simulink model "IEEE24bus_simplified"  (R2019b)
settings: Solver=ode23tb  StartTime=0.0  StopTime=100  MaxStep=1/60  RelTol=1e-4  AbsTol=1e-3  EnableMultiTasking=on
PreLoadFcn:
  | RTS96_data
values from neighbouring files (symbols this model uses):
  Efmax = 5    [IEEE24_bus.m]    (also in IEEE24bus_simplified_benchmark.m)
  Efmin = -5    [IEEE24_bus.m]    (also in IEEE24bus_simplified_benchmark.m)
  EXc_sys = [     0.06  25  0.2    0.0505  0.5685   0 0   0.091  0.35 ... (first row only)    [IEEE24bus_simplified_benchmark.m]
  FH1 = 12    [IEEE24bus_simplified_benchmark.m]
  FI1 = .9    (= 0.9)    [IEEE24bus_simplified_benchmark.m]
  FL1 = .1    (= 0.1)    [IEEE24bus_simplified_benchmark.m]
  KH1 = 100    [IEEE24bus_simplified_benchmark.m]
  KI1 = 1    [IEEE24_bus.m]    (also in IEEE24bus_simplified_benchmark.m = 20)
  KL1 = 10    [IEEE24bus_simplified_benchmark.m]
undefined symbols (not defined in the file or in its folder): D1, Delta
libraries: powerlib x157, sps_avr x11, powerlib_extras x1
(part 1 of 3)
settings Model: Creator=bx6353  LastModifiedBy=mingj
settings SolverCC: AutoScaleAbsTol=off  ZeroCrossControl=DisableAll
settings DataIOCC: InitialState=xFinal  LimitDataPoints=on  SaveFinalState=on  SaveFormat=Array  SignalLoggingSaveFormat=ModelDataLogs  ReturnWorkspaceOutputs=off
settings OptimizationCC: ExpressionDepthLimit=2147483647  InitFltsAndDblsToZero=on  LifeSpan=inf
settings DebuggingCC: SaveWithParameterizedLinksMsg=none  UnderspecifiedInitializationDetection=Classic  MergeDetectMultiDrivingBlocksExec=none  SignalResolutionControl=TryResolveAllWithWarning  SolverPrmCheckMsg=warning  MultiTaskDSMMsg=warning  MultiTaskCondExecSysMsg=none  FcnCallInpInsideContextMsg=warning  UnconnectedInputMsg=none  UnconnectedOutputMsg=none  UnconnectedLineMsg=none  StateNameClashWarn=warning  StrictBusMsg=ErrorOnBusTreatedAsVector  SFUnexpectedBacktrackingDiag=warning  SFNoUnconditionalDefaultTransitionDiag=warning  SFExecutionAtInitializationDiag=none  ArithmeticOperatorsInVariantConditions=warning
settings HardwareCC: ProdBitPerPointer=32  ProdBitPerSizeT=32  ProdBitPerPtrDiffT=32  ProdLargestAtomicFloat=None  ProdIntDivRoundTo=Undefined  ProdEndianess=Unspecified  ProdWordSize=32  ProdHWDeviceType=32-bit Generic
settings ModelReferenceCC: PropagateSignalLabelsOutOfModel=off
settings SFSimCC: SimUseLocalCustomCode=off  CustomCodeUndefinedFunction=UseInterfaceOnly
settings RTWCC: RTWUseLocalCustomCode=off
settings CodeAppCC: StateflowObjectComments=on
settings GRTTargetCC: TargetFcnLib=ansi_tfl_tmw.mat  TargetLangStandard=C89/C90 (ANSI)  GeneratePreprocessorConditionals=Disable all  CombineOutputUpdateFcns=off  GRTInterface=on
settings ConfigComp: CovMetricSettings=dw  CovHtmlReporting=on  CovSaveCumulativeToWorkspaceVar=on  CovSaveSingleToWorkspaceVar=on  CovExternalEMLEnable=off
settings SimscapeCC: SimscapeNormalizeSystem=off

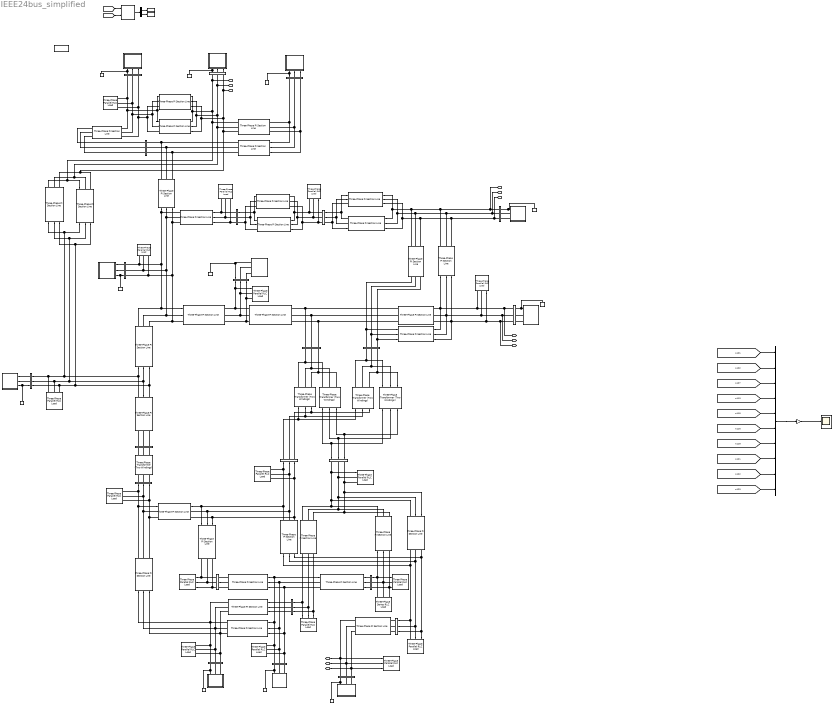
== system IEEE24bus_simplified ==
  101 : Subsystem
  102 : Subsystem
  107 : Subsystem
  113 : Subsystem
  114 : Subsystem
  115 : Subsystem
  116 : Subsystem
  118 : Subsystem
  121 : Subsystem
  122 : Subsystem
  123 : Subsystem
  3-phase  Instantaneous  Active & Reactive Power : powerlib_extras/Measurements/3-phase  Instantaneous  Active & Reactive Power
      settings: SourceProductName=Simscape Electrical  SourceProductBaseCode=PS
  A1 : powerlib/Elements/Three-Phase PI Section Line  LConnTagsString=a|b|c  RConnTagsString=A|B|C  Frequency=60  Resistances=[ 0.003*(138e3)^2/100e6*[1 3]]  Inductances=[ 0.014*(138e3)^2/(120*pi*100e6)*[1 3]]  Capacitances=[0.461*100e6/(120*pi*(138e3)^2)*[1 1/3]]  Length=1
      settings: SourceProductName=Simscape Electrical
  A10 : powerlib/Elements/Three-Phase PI Section Line  LConnTagsString=a|b|c  RConnTagsString=A|B|C  Frequency=60  Resistances=[ 0.014*(138e3)^2/100e6*[1 3]]  Inductances=[ 0.061*(138e3)^2/(120*pi*100e6)*[1 3]]  Capacitances=[2.459*100e6/(120*pi*((138e3)^2))*[1 1/3]]  Length=1
      settings: SourceProductName=Simscape Electrical
  A11 : powerlib/Elements/Three-Phase PI Section Line  LConnTagsString=a|b|c  RConnTagsString=A|B|C  Frequency=60  Resistances=[ 0.016*(138e3)^2/100e6*[1 3]]  Inductances=[ 0.061*(138e3)^2/(120*pi*100e6) *[1 3]]  Capacitances=[0.017*100e6/(120*pi*(138e3)^2) *[1 1/3]]  Length=1
      settings: SourceProductName=Simscape Electrical
  A12-1 : powerlib/Elements/Three-Phase PI Section Line  LConnTagsString=a|b|c  RConnTagsString=A|B|C  Frequency=60  Resistances=[ 0.043*(138e3)^2/100e6 *[1 3]]  Inductances="[ 0.165*(138e3)^2/(120*pi*100e6)  *[1 3]]"  Capacitances=[0.045*100e6/(120*pi*(138e3)^2) *[1 1/3]]  Length=1
      settings: SourceProductName=Simscape Electrical
  A13-2 : powerlib/Elements/Three-Phase PI Section Line  LConnTagsString=a|b|c  RConnTagsString=A|B|C  Frequency=60  Resistances=[ 0.043*(138E3)^2/100E6*[1 3]]  Inductances=[ 0.165*(138e3)^2/(120*pi*100e6)*[1 3]]  Capacitances=[0.045*100e6/(120*pi*(138e3)^2)*[1 1/3]]  Length=1
      settings: SourceProductName=Simscape Electrical
  A{7,14..17} (5 alike) : powerlib/Elements/Three-Phase Transformer (Two Windings)  Winding1Connection=Y  Winding2Connection=Y  CoreType=Three single-phase transformers  SetSaturation=off  Hysteresis=off  DataFile='hysteresis'  SetInitialFlux=off  Measurements=None  UNITS=pu  NominalPower=[ 100e6 , 60 ]  Winding1=[ 230e3 , 0.001 , 0.084/2 ]  Winding2="[ 138e3 , 0.001 , 0.084/2  ]"  Rm=500  Lm=500  L0=0.5  Saturation=[ 0,0 ; 0.0024,1.2 ; 1.0,1.52 ]  InitialFluxes=[ 0.8 , -0.8 , 0.7 ]  BreakLoop=off  DiscreteSolver=Trapezoidal iterative  DataType=off  TransfoNumber=0
      settings: SourceProductName=Simscape Electrical
  A18 : powerlib/Elements/Three-Phase PI Section Line  LConnTagsString=a|b|c  RConnTagsString=A|B|C  Frequency=60  Resistances=[ 0.006*(230e3)^2/100e6*[1 3]]  Inductances=[ 0.048*(230e3)^2/(120*pi*100e6)*[1 3]]  Capacitances=[0.1*100e6/(120*pi*(230e3)^2)*[1 1/3]]  Length=1
      settings: SourceProductName=Simscape Electrical
  A19 : powerlib/Elements/Three-Phase PI Section Line  LConnTagsString=a|b|c  RConnTagsString=A|B|C  Frequency=60  Resistances=[ 0.005*(230e3)^2/(100e6)*[1 3]]  Inductances=[ 0.042*(230e3)^2/(120*pi*100e6)*[1 3]]  Capacitances=[0.088*100e6/(120*pi*(230e3)^2)*[1 1/3]]  Length=1
      settings: SourceProductName=Simscape Electrical
  A2 : powerlib/Elements/Three-Phase PI Section Line  LConnTagsString=a|b|c  RConnTagsString=A|B|C  Frequency=60  Resistances=[ 0.055*(138e3)^2/100e6*[1 3]]  Inductances=[ 0.211*(138e3)^2/(120*pi*100e6)*[1 3]]  Capacitances=[0.057*100e6/(120*pi*(138e3)^2) *[1 1/3]]  Length=1
      settings: SourceProductName=Simscape Electrical
  A20 : powerlib/Elements/Three-Phase PI Section Line  LConnTagsString=a|b|c  RConnTagsString=A|B|C  Frequency=60  Resistances=[ 0.006*(230e3)^2/100e6*[1 3]]  Inductances=[ 0.048*(230e3)^2/(120*pi*100e6)*[1 3]]  Capacitances=[0.1*100e6/(120*pi*(230e3)^2)*[1 1/3]]  Length=1
      settings: SourceProductName=Simscape Electrical
  A21 : powerlib/Elements/Three-Phase PI Section Line  LConnTagsString=a|b|c  RConnTagsString=A|B|C  Frequency=60  Resistances=[ 0.012*(230e3)^2/100e6*[1 3]]  Inductances=[ 0.097*(230e3)^2/(120*pi*100e6)*[1 3]]  Capacitances=[0.203*100e6/(120*pi*(230e3)^2)*[1 1/3]]  Length=1
      settings: SourceProductName=Simscape Electrical
  A22 : powerlib/Elements/Three-Phase PI Section Line  LConnTagsString=a|b|c  RConnTagsString=A|B|C  Frequency=60  Resistances=[ 0.011*(230e3)^2/100e6*[1 3]]  Inductances=[ 0.087*(230e3)^2/(120*pi*100e6) *[1 3]]  Capacitances=[0.182*100e6/(120*pi*(230e3)^2) *[1 1/3]]  Length=1
      settings: SourceProductName=Simscape Electrical
  A23 : powerlib/Elements/Three-Phase PI Section Line  LConnTagsString=a|b|c  RConnTagsString=A|B|C  Frequency=60  Resistances=[ 0.005*(230e3)^2/100e6*[1 3]]  Inductances=[ 0.059*(230e3)^2/(120*pi*100e6) *[1 3]]  Capacitances=[0.082*(100e6)/(120*pi*(230e3)^2)*[1 1/3]]  Length=1
      settings: SourceProductName=Simscape Electrical
  A24 : powerlib/Elements/Three-Phase PI Section Line  LConnTagsString=a|b|c  RConnTagsString=A|B|C  Frequency=60  Resistances=[ 0.002*(230e3)^2/100e6*[1 3]]  Inductances="[ 0.017*(230e3)^2/(120*pi*100e6)  *[1 3]]"  Capacitances=[0.036*100e6/(120*pi*(230e3)^2) *[1 1/3]]  Length=1
      settings: SourceProductName=Simscape Electrical
  A25-1 : powerlib/Elements/Three-Phase PI Section Line  LConnTagsString=a|b|c  RConnTagsString=A|B|C  Frequency=60  Resistances=[ 0.006*(230e3)^2/100e6*[1 3]]  Inductances=[ 0.049*(230e3)^2/(120*pi*100e6)*[1 3]]  Capacitances=[0.103*(100e6)/(120*pi*(230e3)^2)*[1 1/3]]  Length=1
      settings: SourceProductName=Simscape Electrical
  A25-2 : powerlib/Elements/Three-Phase PI Section Line  LConnTagsString=a|b|c  RConnTagsString=A|B|C  Frequency=60  Resistances=[ 0.006*(230e3)^2/100e6 *[1 3]]  Inductances=[ 0.049*(230e3)^2/(120*pi*100e6)*[1 3]]  Capacitances=[0.103*(100e6)/(120*pi*(230e3)^2)*[1 1/3]]  Length=1
      settings: SourceProductName=Simscape Electrical
  A26 : powerlib/Elements/Three-Phase PI Section Line  LConnTagsString=a|b|c  RConnTagsString=A|B|C  Frequency=60  Resistances=[ 0.007*(230e3)^2/100e6*[1 3]]  Inductances=[ 0.052*(230e3)^2/(120*pi*100e6) *[1 3]]  Capacitances=[0.109*100e6/(120*pi*(230e3)^2)*[1 1/3]]  Length=1
      settings: SourceProductName=Simscape Electrical
  A27 : powerlib/Elements/Three-Phase PI Section Line  LConnTagsString=a|b|c  RConnTagsString=A|B|C  Frequency=60  Resistances=[ 0.003*(230e3)^2/100e6*[1 3]]  Inductances=[ 0.026*(230e3)^2/(120*pi*100e6) *[1 3]]  Capacitances=[0.055*100e6/(120*pi*(230e3)^2) *[1 1/3]]  Length=1
      settings: SourceProductName=Simscape Electrical
  A28 : powerlib/Elements/Three-Phase PI Section Line  LConnTagsString=a|b|c  RConnTagsString=A|B|C  Frequency=60  Resistances=[ 0.003*(230e3)^2/100e6*[1 3]]  Inductances=[ 0.023*(230e3)^2/(120*pi*100e6)*[1 3]]  Capacitances=[0.049*100e6/(120*pi*(230e3)^2)*[1 1/3]]  Length=1
      settings: SourceProductName=Simscape Electrical
  A29 : powerlib/Elements/Three-Phase PI Section Line  LConnTagsString=a|b|c  RConnTagsString=A|B|C  Frequency=60  Resistances=[ 0.002*(230e3)^2/100e6*[1 3]]  Inductances=[ 0.014*(230e3)^2/(120*pi*100e6)*[1 3]]  Capacitances=[0.030*100e6/(120*pi*(230e3)^2)*[1 1/3]]  Length=1
      settings: SourceProductName=Simscape Electrical
  A3 : powerlib/Elements/Three-Phase PI Section Line  LConnTagsString=a|b|c  RConnTagsString=A|B|C  Frequency=60  Resistances=[0.022*(138e3)^2/100e6*[1 3]]  Inductances=[0.085*(138e3)^2/(120*pi*100e6)*[1 3]]  Capacitances=[0.023*100e6/(120*pi*(138e3)^2)*[1 1/3]]  Length=1
      settings: SourceProductName=Simscape Electrical
  A30 : powerlib/Elements/Three-Phase PI Section Line  LConnTagsString=a|b|c  RConnTagsString=A|B|C  Frequency=60  Resistances=[ 0.014*(230e3)^2/100e6 *[1 3]]  Inductances=[ 0.105*(230e3)^2/(120*pi*100e6) *[1 3]]  Capacitances=[0.221*100e6/(120*pi*(230e3)^2)*[1 1/3]]  Length=1
      settings: SourceProductName=Simscape Electrical
  A31-1 : powerlib/Elements/Three-Phase PI Section Line  LConnTagsString=a|b|c  RConnTagsString=A|B|C  Frequency=60  Resistances=[ 0.003*(230e3)^2/100e6*[1 3]]  Inductances=[ 0.026*(230e3)^2/(120*pi*100e6)*[1 3]]  Capacitances=[0.055*100e6/(120*pi*(230e3)^2)*[1 1/3]]  Length=1
      settings: SourceProductName=Simscape Electrical
  A31-2 : powerlib/Elements/Three-Phase PI Section Line  LConnTagsString=a|b|c  RConnTagsString=A|B|C  Frequency=60  Resistances=[ 0.003*(230e3)^2/100e6*[1 3]]  Inductances=[ 0.026*(230e3)^2/(120*pi*100e6) *[1 3]]  Capacitances=[0.055*100e6/(120*pi*(230e3)^2) *[1 1/3]]  Length=1
      settings: SourceProductName=Simscape Electrical
  A32-2 : powerlib/Elements/Three-Phase PI Section Line  LConnTagsString=a|b|c  RConnTagsString=A|B|C  Frequency=60  Resistances=[ 0.005*(230e3)^2/100e6 *[1 3]]  Inductances=[ 0.040*(230e3)^2/(120*pi*100e6)*[1 3]]  Capacitances=[0.083*100e6/(120*pi*(230e3)^2) *[1 1/3]]  Length=1
      settings: SourceProductName=Simscape Electrical
  A32-3 : powerlib/Elements/Three-Phase PI Section Line  LConnTagsString=a|b|c  RConnTagsString=A|B|C  Frequency=60  Resistances=[ 0.005*(230e3)^2/100e6*[1 3]]  Inductances=[ 0.040*(230e3)^2/(120*pi*100e6) *[1 3]]  Capacitances=[0.083*100e6/(120*pi*(230e3)^2)*[1 1/3]]  Length=1
      settings: SourceProductName=Simscape Electrical
  A33-1 : powerlib/Elements/Three-Phase PI Section Line  LConnTagsString=a|b|c  RConnTagsString=A|B|C  Frequency=60  Resistances=[ 0.003*(230e3)^2/100e6*[1 3]]  Inductances=[ 0.022*(230e3)^2/(120*pi*100e6) *[1 3]]  Capacitances=[0.046*100e6/(120*pi*(230e3)^2) *[1 1/3]]  Length=1
      settings: SourceProductName=Simscape Electrical
  A33-2 : powerlib/Elements/Three-Phase PI Section Line  LConnTagsString=a|b|c  RConnTagsString=A|B|C  Frequency=60  Resistances=[ 0.003*(230e3)^2/100e6*[1 3]]  Inductances=[ 0.022*(230e3)^2/(120*pi*100e6) *[1 3]]  Capacitances=[0.046*100e6/(120*pi*(230e3)^2) *[1 1/3]]  Length=1
      settings: SourceProductName=Simscape Electrical
  A34 : powerlib/Elements/Three-Phase PI Section Line  LConnTagsString=a|b|c  RConnTagsString=A|B|C  Frequency=60  Resistances=[ 0.009*(230e3)^2/100e6*[1 3]]  Inductances=[ 0.068*(230e3)^2/(120*pi*100e6) *[1 3]]  Capacitances=[0.142*100e6/(120*pi*(230e3)^2)*[1 1/3]]  Length=1
      settings: SourceProductName=Simscape Electrical
  A4 : powerlib/Elements/Three-Phase PI Section Line  LConnTagsString=a|b|c  RConnTagsString=A|B|C  Frequency=60  Resistances=[ 0.033*(138e3)^2/100e6 *[1 3]]  Inductances="[ 0.127*(138e3)^2/(120*pi*100e6)  *[1 3]]"  Capacitances=[0.034*100e6/(120*pi*(138e3)^2) *[1 1/3]]  Length=1
      settings: SourceProductName=Simscape Electrical
  A5 : powerlib/Elements/Three-Phase PI Section Line  LConnTagsString=a|b|c  RConnTagsString=A|B|C  Frequency=60  Resistances=[ 0.050*(138e3)^2/100e6*[1 3]]  Inductances="[ 0.192*(138e3)^2/(120*pi*100e6)  *[1 3]]"  Capacitances=[0.052*100e6/(120*pi*(138e3)^2)*[1 3]]  Length=1
      settings: SourceProductName=Simscape Electrical
  A6 : powerlib/Elements/Three-Phase PI Section Line  LConnTagsString=a|b|c  RConnTagsString=A|B|C  Frequency=60  Resistances=[ 0.031*(138e3)^2/100e6 *[1 3]]  Inductances=[ 0.119*(138e3)^2/(120*pi*100e6) *[1 3]]  Capacitances=[0.032*100e6/(120*pi*(138e3)^2)*[1 3]]  Length=1
      settings: SourceProductName=Simscape Electrical
  A8 : powerlib/Elements/Three-Phase PI Section Line  LConnTagsString=a|b|c  RConnTagsString=A|B|C  Frequency=60  Resistances=[ 0.027*(138e3)^2/100e6*[1 3]]  Inductances=[ 0.104*(138e3)^2/(120*pi*100e6) *[1 3]]  Capacitances=[0.028*100e6/(120*pi*(138e3)^2) *[1 3]]  Length=1
      settings: SourceProductName=Simscape Electrical
  A9 : powerlib/Elements/Three-Phase PI Section Line  LConnTagsString=a|b|c  RConnTagsString=A|B|C  Frequency=60  Resistances=[ 0.023*(138e3)^2/100e6 *[1 3]]  Inductances="[ 0.088*(138e3)^2/(120*pi*100e6)  *[1 3]]"  Capacitances=[0.024*100e6/(120*pi*(138e3)^2) *[1 3]]  Length=1
      settings: SourceProductName=Simscape Electrical
  B101 : powerlib/Measurements/Three-Phase V-I Measurement  VoltageMeasurement=phase-to-phase  SetLabelV=on  LabelV=Vabc_B101  Vpu=off  VpuLL=on  CurrentMeasurement=yes  SetLabelI=on  LabelI=Iabc_B101  Ipu=on  Pbase=100e6  Vbase=138e3  OutputType=Complex  PhasorSimulation=on  PSBequivalent=0
      settings: SourceProductName=Simscape Electrical
  B102 : powerlib/Measurements/Three-Phase V-I Measurement  VoltageMeasurement=phase-to-ground  SetLabelV=on  LabelV=Vabc_B102  Vpu=on  VpuLL=off  CurrentMeasurement=yes  SetLabelI=on  LabelI=Iabc_B102  Ipu=on  Pbase=100e6  Vbase=138e3  OutputType=Complex  PhasorSimulation=on  PSBequivalent=0
      settings: SourceProductName=Simscape Electrical
  B103 : powerlib/Measurements/Three-Phase V-I Measurement  VoltageMeasurement=no  SetLabelV=on  LabelV=Vabc_B103  Vpu=on  VpuLL=off  CurrentMeasurement=no  SetLabelI=on  LabelI=Iabc_B103  Ipu=on  Pbase=100e6  Vbase=138e3  OutputType=Complex  PhasorSimulation=on  PSBequivalent=0
      settings: SourceProductName=Simscape Electrical
  B104 : powerlib/Measurements/Three-Phase V-I Measurement  VoltageMeasurement=no  SetLabelV=on  LabelV=Vabc_B104  Vpu=on  VpuLL=off  CurrentMeasurement=no  SetLabelI=on  LabelI=Iabc_B104  Ipu=on  Pbase=100e6  Vbase=138e3  OutputType=Complex  PhasorSimulation=on  PSBequivalent=0
      settings: SourceProductName=Simscape Electrical
  B105 : powerlib/Measurements/Three-Phase V-I Measurement  VoltageMeasurement=no  SetLabelV=on  LabelV=Vabc_B105  Vpu=on  VpuLL=off  CurrentMeasurement=no  SetLabelI=on  LabelI=Iabc_B105  Ipu=on  Pbase=100e6  Vbase=138e3  OutputType=Complex  PhasorSimulation=on  PSBequivalent=0
      settings: SourceProductName=Simscape Electrical
  B106 : powerlib/Measurements/Three-Phase V-I Measurement  VoltageMeasurement=no  SetLabelV=on  LabelV=Vabc_B106  Vpu=on  VpuLL=off  CurrentMeasurement=no  SetLabelI=on  LabelI=Iabc_B106  Ipu=on  Pbase=100e6  Vbase=138e3  OutputType=Complex  PhasorSimulation=on  PSBequivalent=0
      settings: SourceProductName=Simscape Electrical
  B107 : powerlib/Measurements/Three-Phase V-I Measurement  VoltageMeasurement=phase-to-ground  SetLabelV=on  LabelV=Vabc_B107  Vpu=on  VpuLL=off  CurrentMeasurement=yes  SetLabelI=on  LabelI=Iabc_B107  Ipu=on  Pbase=100e6  Vbase=138e3  OutputType=Complex  PhasorSimulation=on  PSBequivalent=0
      settings: SourceProductName=Simscape Electrical
  B108 : powerlib/Measurements/Three-Phase V-I Measurement  VoltageMeasurement=no  SetLabelV=on  LabelV=Vabc_B108  Vpu=on  VpuLL=off  CurrentMeasurement=no  SetLabelI=on  LabelI=Iabc_B108  Ipu=on  Pbase=100e6  Vbase=138e3  OutputType=Complex  PhasorSimulation=on  PSBequivalent=0
      settings: SourceProductName=Simscape Electrical
  B109 : powerlib/Measurements/Three-Phase V-I Measurement  VoltageMeasurement=no  SetLabelV=on  LabelV=Vabc_B109  Vpu=on  VpuLL=off  CurrentMeasurement=no  SetLabelI=on  LabelI=Iabc_B109  Ipu=on  Pbase=100e6  Vbase=138e3  OutputType=Complex  PhasorSimulation=on  PSBequivalent=0
      settings: SourceProductName=Simscape Electrical
  B110 : powerlib/Measurements/Three-Phase V-I Measurement  VoltageMeasurement=no  SetLabelV=on  LabelV=Vabc_B110  Vpu=on  VpuLL=off  CurrentMeasurement=no  SetLabelI=on  LabelI=Iabc_B110  Ipu=on  Pbase=100e6  Vbase=138e3  OutputType=Complex  PhasorSimulation=on  PSBequivalent=0
      settings: SourceProductName=Simscape Electrical
  B111 : powerlib/Measurements/Three-Phase V-I Measurement  VoltageMeasurement=no  SetLabelV=on  LabelV=Vabc_B111  Vpu=on  VpuLL=off  CurrentMeasurement=no  SetLabelI=on  LabelI=Iabc_B111  Ipu=on  Pbase=100e6  Vbase=230e3  OutputType=Complex  PhasorSimulation=on  PSBequivalent=0
      settings: SourceProductName=Simscape Electrical
  B112 : powerlib/Measurements/Three-Phase V-I Measurement  VoltageMeasurement=no  SetLabelV=on  LabelV=Vabc_B112  Vpu=on  VpuLL=off  CurrentMeasurement=no  SetLabelI=on  LabelI=Iabc_B112  Ipu=on  Pbase=100e6  Vbase=230e3  OutputType=Complex  PhasorSimulation=on  PSBequivalent=0
      settings: SourceProductName=Simscape Electrical
  B113 : powerlib/Measurements/Three-Phase V-I Measurement  VoltageMeasurement=phase-to-ground  SetLabelV=on  LabelV=Vabc_B113  Vpu=on  VpuLL=off  CurrentMeasurement=yes  SetLabelI=on  LabelI=Iabc_B113  Ipu=on  Pbase=100e6  Vbase=230e3  OutputType=Complex  PhasorSimulation=on  PSBequivalent=0
      settings: SourceProductName=Simscape Electrical
  B114 : powerlib/Measurements/Three-Phase V-I Measurement  VoltageMeasurement=phase-to-ground  SetLabelV=on  LabelV=Vabc_B114  Vpu=on  VpuLL=off  CurrentMeasurement=yes  SetLabelI=on  LabelI=Iabc_B114  Ipu=on  Pbase=100e6  Vbase=230e3  OutputType=Complex  PhasorSimulation=on  PSBequivalent=0
      settings: SourceProductName=Simscape Electrical
  B115 : powerlib/Measurements/Three-Phase V-I Measurement  VoltageMeasurement=phase-to-ground  SetLabelV=on  LabelV=Vabc_B115  Vpu=on  VpuLL=off  CurrentMeasurement=yes  SetLabelI=on  LabelI=Iabc_B115  Ipu=on  Pbase=100e6  Vbase=230e3  OutputType=Complex  PhasorSimulation=on  PSBequivalent=0
      settings: SourceProductName=Simscape Electrical
  B116 : powerlib/Measurements/Three-Phase V-I Measurement  VoltageMeasurement=phase-to-ground  SetLabelV=on  LabelV=Vabc_B116  Vpu=on  VpuLL=off  CurrentMeasurement=yes  SetLabelI=on  LabelI=Iabc_B116  Ipu=on  Pbase=100e6  Vbase=230e3  OutputType=Complex  PhasorSimulation=on  PSBequivalent=0
      settings: SourceProductName=Simscape Electrical
  B117 : powerlib/Measurements/Three-Phase V-I Measurement  VoltageMeasurement=no  SetLabelV=on  LabelV=Vabc_B117  Vpu=on  VpuLL=off  CurrentMeasurement=no  SetLabelI=on  LabelI=Iabc_B117  Ipu=on  Pbase=100e6  Vbase=230e3  OutputType=Complex  PhasorSimulation=on  PSBequivalent=0
      settings: SourceProductName=Simscape Electrical
  B118 : powerlib/Measurements/Three-Phase V-I Measurement  VoltageMeasurement=phase-to-ground  SetLabelV=on  LabelV=Vabc_B118  Vpu=on  VpuLL=off  CurrentMeasurement=yes  SetLabelI=on  LabelI=Iabc_B118  Ipu=on  Pbase=100e6  Vbase=230e3  OutputType=Complex  PhasorSimulation=on  PSBequivalent=0
      settings: SourceProductName=Simscape Electrical
  B119 : powerlib/Measurements/Three-Phase V-I Measurement  VoltageMeasurement=no  SetLabelV=on  LabelV=Vabc_B119  Vpu=on  VpuLL=off  CurrentMeasurement=no  SetLabelI=on  LabelI=Iabc_B119  Ipu=on  Pbase=100e6  Vbase=230e3  OutputType=Complex  PhasorSimulation=on  PSBequivalent=0
      settings: SourceProductName=Simscape Electrical
  B120 : powerlib/Measurements/Three-Phase V-I Measurement  VoltageMeasurement=no  SetLabelV=on  LabelV=Vabc_B120  Vpu=on  VpuLL=off  CurrentMeasurement=no  SetLabelI=on  LabelI=Iabc_B120  Ipu=on  Pbase=100e6  Vbase=230e3  OutputType=Complex  PhasorSimulation=on  PSBequivalent=0
      settings: SourceProductName=Simscape Electrical
  B121 : powerlib/Measurements/Three-Phase V-I Measurement  VoltageMeasurement=phase-to-ground  SetLabelV=on  LabelV=Vabc_B121  Vpu=on  VpuLL=off  CurrentMeasurement=yes  SetLabelI=on  LabelI=Iabc_B121  Ipu=on  Pbase=100e6  Vbase=230e3  OutputType=Complex  PhasorSimulation=on  PSBequivalent=0
      settings: SourceProductName=Simscape Electrical
  B122 : powerlib/Measurements/Three-Phase V-I Measurement  VoltageMeasurement=phase-to-ground  SetLabelV=on  LabelV=Vabc_B122  Vpu=on  VpuLL=off  CurrentMeasurement=yes  SetLabelI=on  LabelI=Iabc_B122  Ipu=on  Pbase=100e6  Vbase=230e3  OutputType=Complex  PhasorSimulation=on  PSBequivalent=0
      settings: SourceProductName=Simscape Electrical
  B123 : powerlib/Measurements/Three-Phase V-I Measurement  VoltageMeasurement=phase-to-ground  SetLabelV=on  LabelV=Vabc_B123  Vpu=on  VpuLL=off  CurrentMeasurement=yes  SetLabelI=on  LabelI=Iabc_B123  Ipu=on  Pbase=100e6  Vbase=230e3  OutputType=Complex  PhasorSimulation=on  PSBequivalent=0
      settings: SourceProductName=Simscape Electrical
  B124 : powerlib/Measurements/Three-Phase V-I Measurement  VoltageMeasurement=no  SetLabelV=on  LabelV=Vabc_B124  Vpu=on  VpuLL=off  CurrentMeasurement=no  SetLabelI=on  LabelI=Iabc_B124  Ipu=on  Pbase=100e6  Vbase=230e3  OutputType=Complex  PhasorSimulation=on  PSBequivalent=0
      settings: SourceProductName=Simscape Electrical
  Demux : Demux  Outputs=2
  L101 : powerlib/Elements/Three-Phase Parallel RLC Load  LConnTagsString=A|B|C  Configuration=Y (grounded)  NominalVoltage=(138000)*0.997799  Vabc=[1e3 1e3 1e3]  Vabcp=[1e3 1e3 1e3]  NominalFrequency=60  UnbalancedPower=off  ActivePower=108e6  InductivePower=22e6  CapacitivePower=0  Pabc=[10e3 9e3 11e3]  QLabc=[100 90 110]  QCabc=[100 90 110]  Pabcp=[10e3 9e3 11e3]  QLabcp=[100 90 110]  QCabcp=[100 90 110]  Measurements=None  LoadType=constant PQ
      settings: SourceProductName=Simscape Electrical
  L102 : powerlib/Elements/Three-Phase Parallel RLC Load  LConnTagsString=A|B|C  Configuration=Y (grounded)  NominalVoltage=(138000)*1.00093  Vabc=[1e3 1e3 1e3]  Vabcp=[1e3 1e3 1e3]  NominalFrequency=60  UnbalancedPower=off  ActivePower=97e6  InductivePower=20e6  CapacitivePower=0  Pabc=[10e3 9e3 11e3]  QLabc=[100 90 110]  QCabc=[100 90 110]  Pabcp=[10e3 9e3 11e3]  QLabcp=[100 90 110]  QCabcp=[100 90 110]  Measurements=None  LoadType=constant PQ
      settings: SourceProductName=Simscape Electrical
  L103 : powerlib/Elements/Three-Phase Parallel RLC Load  LConnTagsString=A|B|C  Configuration=Y (grounded)  NominalVoltage=(127400)*1  Vabc=[1e3 1e3 1e3]  Vabcp=[1e3 1e3 1e3]  NominalFrequency=60  UnbalancedPower=off  ActivePower=180e6  InductivePower=37e6  CapacitivePower=0  Pabc=[10e3 9e3 11e3]  QLabc=[100 90 110]  QCabc=[100 90 110]  Pabcp=[10e3 9e3 11e3]  QLabcp=[100 90 110]  QCabcp=[100 90 110]  Measurements=None  LoadType=constant PQ
      settings: SourceProductName=Simscape Electrical
  L104 : powerlib/Elements/Three-Phase Parallel RLC Load  LConnTagsString=A|B|C  Configuration=Y (grounded)  NominalVoltage=(131169)*1  Vabc=[1e3 1e3 1e3]  Vabcp=[1e3 1e3 1e3]  NominalFrequency=60  UnbalancedPower=off  ActivePower=74e6  InductivePower=15e6  CapacitivePower=0  Pabc=[10e3 9e3 11e3]  QLabc=[100 90 110]  QCabc=[100 90 110]  Pabcp=[10e3 9e3 11e3]  QLabcp=[100 90 110]  QCabcp=[100 90 110]  Measurements=None  LoadType=constant PQ
      settings: SourceProductName=Simscape Electrical
  L105 : powerlib/Elements/Three-Phase Parallel RLC Load  LConnTagsString=A|B|C  Configuration=Y (grounded)  NominalVoltage=(137498)*1  Vabc=[1e3 1e3 1e3]  Vabcp=[1e3 1e3 1e3]  NominalFrequency=60  UnbalancedPower=off  ActivePower=71e6  InductivePower=14e6  CapacitivePower=0  Pabc=[10e3 9e3 11e3]  QLabc=[100 90 110]  QCabc=[100 90 110]  Pabcp=[10e3 9e3 11e3]  QLabcp=[100 90 110]  QCabcp=[100 90 110]  Measurements=None  LoadType=constant PQ
      settings: SourceProductName=Simscape Electrical
  L106 : powerlib/Elements/Three-Phase Parallel RLC Load  LConnTagsString=A|B|C  Configuration=Y (grounded)  NominalVoltage=(151009)*1  Vabc=[1e3 1e3 1e3]  Vabcp=[1e3 1e3 1e3]  NominalFrequency=60  UnbalancedPower=off  ActivePower=136e6  InductivePower=28e6  CapacitivePower=0  Pabc=[10e3 9e3 11e3]  QLabc=[100 90 110]  QCabc=[100 90 110]  Pabcp=[10e3 9e3 11e3]  QLabcp=[100 90 110]  QCabcp=[100 90 110]  Measurements=None  LoadType=constant PQ
      settings: SourceProductName=Simscape Electrical
  L107 : powerlib/Elements/Three-Phase Parallel RLC Load  LConnTagsString=A|B|C  Configuration=Y (grounded)  NominalVoltage=(138000)*0.974816  Vabc=[1e3 1e3 1e3]  Vabcp=[1e3 1e3 1e3]  NominalFrequency=60  UnbalancedPower=off  ActivePower=125e6  InductivePower=25e6  CapacitivePower=0  Pabc=[10e3 9e3 11e3]  QLabc=[100 90 110]  QCabc=[100 90 110]  Pabcp=[10e3 9e3 11e3]  QLabcp=[100 90 110]  QCabcp=[100 90 110]  Measurements=None  LoadType=constant PQ
      settings: SourceProductName=Simscape Electrical
  L108 : powerlib/Elements/Three-Phase Parallel RLC Load  LConnTagsString=A|B|C  Configuration=Y (grounded)  NominalVoltage=(130970)*0.999997  Vabc=[1e3 1e3 1e3]  Vabcp=[1e3 1e3 1e3]  NominalFrequency=60  UnbalancedPower=off  ActivePower=171e6  InductivePower=35e6  CapacitivePower=0  Pabc=[10e3 9e3 11e3]  QLabc=[100 90 110]  QCabc=[100 90 110]  Pabcp=[10e3 9e3 11e3]  QLabcp=[100 90 110]  QCabcp=[100 90 110]  Measurements=None  LoadType=constant PQ
      settings: SourceProductName=Simscape Electrical
  L109 : powerlib/Elements/Three-Phase Parallel RLC Load  LConnTagsString=A|B|C  Configuration=Y (grounded)  NominalVoltage=(130445)*1  Vabc=[1e3 1e3 1e3]  Vabcp=[1e3 1e3 1e3]  NominalFrequency=60  UnbalancedPower=off  ActivePower=175e6  InductivePower=36e6  CapacitivePower=0  Pabc=[10e3 9e3 11e3]  QLabc=[100 90 110]  QCabc=[100 90 110]  Pabcp=[10e3 9e3 11e3]  QLabcp=[100 90 110]  QCabcp=[100 90 110]  Measurements=None  LoadType=constant PQ
      settings: SourceProductName=Simscape Electrical
  L110 : powerlib/Elements/Three-Phase Parallel RLC Load  LConnTagsString=A|B|C  Configuration=Y (grounded)  NominalVoltage=(141150)*0.999999  Vabc=[1e3 1e3 1e3]  Vabcp=[1e3 1e3 1e3]  NominalFrequency=60  UnbalancedPower=off  ActivePower=195e6  InductivePower=40e6  CapacitivePower=0  Pabc=[10e3 9e3 11e3]  QLabc=[100 90 110]  QCabc=[100 90 110]  Pabcp=[10e3 9e3 11e3]  QLabcp=[100 90 110]  QCabcp=[100 90 110]  Measurements=None  LoadType=constant PQ
      settings: SourceProductName=Simscape Electrical
  L113 : powerlib/Elements/Three-Phase Parallel RLC Load  LConnTagsString=A|B|C  Configuration=Y (grounded)  NominalVoltage=(230000)*0.974192  Vabc=[1e3 1e3 1e3]  Vabcp=[1e3 1e3 1e3]  NominalFrequency=60  UnbalancedPower=off  ActivePower=265e6  InductivePower=54e6  CapacitivePower=0  Pabc=[10e3 9e3 11e3]  QLabc=[100 90 110]  QCabc=[100 90 110]  Pabcp=[10e3 9e3 11e3]  QLabcp=[100 90 110]  QCabcp=[100 90 110]  Measurements=None  LoadType=constant PQ
      settings: SourceProductName=Simscape Electrical
  L114 : powerlib/Elements/Three-Phase Parallel RLC Load  LConnTagsString=A|B|C  Configuration=Y (grounded)  NominalVoltage=(230000)*0.962113  Vabc=[1e3 1e3 1e3]  Vabcp=[1e3 1e3 1e3]  NominalFrequency=60  UnbalancedPower=off  ActivePower=194e6  InductivePower=39e6  CapacitivePower=0  Pabc=[10e3 9e3 11e3]  QLabc=[100 90 110]  QCabc=[100 90 110]  Pabcp=[10e3 9e3 11e3]  QLabcp=[100 90 110]  QCabcp=[100 90 110]  Measurements=None  LoadType=constant PQ
      settings: SourceProductName=Simscape Electrical
  L115 : powerlib/Elements/Three-Phase Parallel RLC Load  LConnTagsString=A|B|C  Configuration=Y (grounded)  NominalVoltage=(230000)*0.95932  Vabc=[1e3 1e3 1e3]  Vabcp=[1e3 1e3 1e3]  NominalFrequency=60  UnbalancedPower=off  ActivePower=317e6  InductivePower=64e6  CapacitivePower=0  Pabc=[10e3 9e3 11e3]  QLabc=[100 90 110]  QCabc=[100 90 110]  Pabcp=[10e3 9e3 11e3]  QLabcp=[100 90 110]  QCabcp=[100 90 110]  Measurements=None  LoadType=constant PQ
      settings: SourceProductName=Simscape Electrical
  L116 : powerlib/Elements/Three-Phase Parallel RLC Load  LConnTagsString=A|B|C  Configuration=Y (grounded)  NominalVoltage=(230000)*0.961708  Vabc=[1e3 1e3 1e3]  Vabcp=[1e3 1e3 1e3]  NominalFrequency=60  UnbalancedPower=off  ActivePower=100e6  InductivePower=20e6  CapacitivePower=0  Pabc=[10e3 9e3 11e3]  QLabc=[100 90 110]  QCabc=[100 90 110]  Pabcp=[10e3 9e3 11e3]  QLabcp=[100 90 110]  QCabcp=[100 90 110]  Measurements=None  LoadType=constant PQ
      settings: SourceProductName=Simscape Electrical
  L118 : powerlib/Elements/Three-Phase Parallel RLC Load  LConnTagsString=A|B|C  Configuration=Y (grounded)  NominalVoltage=(230000)*0.975017  Vabc=[1e3 1e3 1e3]  Vabcp=[1e3 1e3 1e3]  NominalFrequency=60  UnbalancedPower=off  ActivePower=333e6  InductivePower=68e6  CapacitivePower=0  Pabc=[10e3 9e3 11e3]  QLabc=[100 90 110]  QCabc=[100 90 110]  Pabcp=[10e3 9e3 11e3]  QLabcp=[100 90 110]  QCabcp=[100 90 110]  Measurements=None  LoadType=constant PQ
      settings: SourceProductName=Simscape Electrical
  L119 : powerlib/Elements/Three-Phase Parallel RLC Load  LConnTagsString=A|B|C  Configuration=Y (grounded)  NominalVoltage=(221184)*1  Vabc=[1e3 1e3 1e3]  Vabcp=[1e3 1e3 1e3]  NominalFrequency=60  UnbalancedPower=off  ActivePower=181e6  InductivePower=37e6  CapacitivePower=0  Pabc=[10e3 9e3 11e3]  QLabc=[100 90 110]  QCabc=[100 90 110]  Pabcp=[10e3 9e3 11e3]  QLabcp=[100 90 110]  QCabcp=[100 90 110]  Measurements=None  LoadType=constant PQ
      settings: SourceProductName=Simscape Electrical
  L120 : powerlib/Elements/Three-Phase Parallel RLC Load  LConnTagsString=A|B|C  Configuration=Y (grounded)  NominalVoltage=(223684)*1  Vabc=[1e3 1e3 1e3]  Vabcp=[1e3 1e3 1e3]  NominalFrequency=60  UnbalancedPower=off  ActivePower=128e6  InductivePower=26e6  CapacitivePower=0  Pabc=[10e3 9e3 11e3]  QLabc=[100 90 110]  QCabc=[100 90 110]  Pabcp=[10e3 9e3 11e3]  QLabcp=[100 90 110]  QCabcp=[100 90 110]  Measurements=None  LoadType=constant PQ
      settings: SourceProductName=Simscape Electrical
  Load Flow Bus : powerlib/Measurements/Load Flow Bus  LConnTagsString=a  Phases=single  Connectors=on one side  ID=BUS_118  Vbase=230e3  Vref=1.05  Vangle=0  VLF=0.975  VLFb=1  VLFc=1  angleLF=48.06  angleLFb=0  angleLFc=0
      settings: AttributesFormatString=%<ID>\n%<Vbase>V\n%<VLF>pu\n%<angleLF>deg.  SourceProductName=Simscape Electrical
  Load Flow Bus1 : powerlib/Measurements/Load Flow Bus  LConnTagsString=a  Phases=single  Connectors=on one side  ID=BUS_121  Vbase=230e3  Vref=1.05  Vangle=0  VLF=0.9792  VLFb=1  VLFc=1  angleLF=48.86  angleLFb=0  angleLFc=0
      settings: AttributesFormatString=%<ID>\n%<Vbase>V\n%<VLF>pu\n%<angleLF>deg.  SourceProductName=Simscape Electrical
  Load Flow Bus10 : powerlib/Measurements/Load Flow Bus  LConnTagsString=a  Phases=single  Connectors=on one side  ID=BUS_122  Vbase=230e3  Vref=1.05  Vangle=0  VLF=0.9939  VLFb=1  VLFc=1  angleLF=55.21  angleLFb=0  angleLFc=0
      settings: AttributesFormatString=%<ID>\n%<Vbase>V\n%<VLF>pu\n%<angleLF>deg.  SourceProductName=Simscape Electrical
  Load Flow Bus2 : powerlib/Measurements/Load Flow Bus  LConnTagsString=a  Phases=single  Connectors=on one side  ID=BUS_101  Vbase=138e3  Vref=1.035  Vangle=0  VLF=0.9978  VLFb=1  VLFc=1  angleLF=21.25  angleLFb=0  angleLFc=0
      settings: AttributesFormatString=%<ID>\n%<Vbase>V\n%<VLF>pu\n%<angleLF>deg.  SourceProductName=Simscape Electrical
  Load Flow Bus3 : powerlib/Measurements/Load Flow Bus  LConnTagsString=a  Phases=single  Connectors=on one side  ID=BUS_102  Vbase=138e3  Vref=1.035  Vangle=0  VLF=1.001  VLFb=1  VLFc=1  angleLF=21.1  angleLFb=0  angleLFc=0
      settings: AttributesFormatString=%<ID>\n%<Vbase>V\n%<VLF>pu\n%<angleLF>deg.  SourceProductName=Simscape Electrical
  Load Flow Bus4 : powerlib/Measurements/Load Flow Bus  LConnTagsString=a  Phases=single  Connectors=on one side  ID=BUS_107  Vbase=138e3  Vref=1.025  Vangle=0  VLF=0.9748  VLFb=1  VLFc=1  angleLF=21.22  angleLFb=0  angleLFc=0
      settings: AttributesFormatString=%<ID>\n%<Vbase>V\n%<VLF>pu\n%<angleLF>deg.  SourceProductName=Simscape Electrical
  Load Flow Bus5 : powerlib/Measurements/Load Flow Bus  LConnTagsString=a  Phases=single  Connectors=on one side  ID=BUS_115  Vbase=230e3  Vref=1.014  Vangle=0  VLF=0.9593  VLFb=1  VLFc=1  angleLF=42.73  angleLFb=0  angleLFc=0
      settings: AttributesFormatString=%<ID>\n%<Vbase>V\n%<VLF>pu\n%<angleLF>deg.  SourceProductName=Simscape Electrical
  Load Flow Bus6 : powerlib/Measurements/Load Flow Bus  LConnTagsString=a  Phases=single  Connectors=on one side  ID=BUS_114  Vbase=230e3  Vref=.98  Vangle=0  VLF=0.9621  VLFb=1  VLFc=1  angleLF=29.58  angleLFb=0  angleLFc=0
      settings: AttributesFormatString=%<ID>\n%<Vbase>V\n%<VLF>pu\n%<angleLF>deg.  SourceProductName=Simscape Electrical
  Load Flow Bus7 : powerlib/Measurements/Load Flow Bus  LConnTagsString=a  Phases=single  Connectors=on one side  ID=BUS_116  Vbase=230e3  Vref=1.017  Vangle=0  VLF=0.9617  VLFb=1  VLFc=1  angleLF=41.74  angleLFb=0  angleLFc=0
      settings: AttributesFormatString=%<ID>\n%<Vbase>V\n%<VLF>pu\n%<angleLF>deg.  SourceProductName=Simscape Electrical
  Load Flow Bus8 : powerlib/Measurements/Load Flow Bus  LConnTagsString=a  Phases=single  Connectors=on one side  ID=BUS_113  Vbase=230e3  Vref=1.02  Vangle=0  VLF=0.9742  VLFb=1  VLFc=1  angleLF=29.58  angleLFb=0  angleLFc=0
      settings: AttributesFormatString=%<ID>\n%<Vbase>V\n%<VLF>pu\n%<angleLF>deg.  SourceProductName=Simscape Electrical
  Load Flow Bus9 : powerlib/Measurements/Load Flow Bus  LConnTagsString=a  Phases=single  Connectors=on one side  ID=BUS_123  Vbase=230e3  Vref=1.05  Vangle=0  VLF=0.9824  VLFb=1  VLFc=1  angleLF=41.99  angleLFb=0  angleLFc=0
      settings: AttributesFormatString=%<ID>\n%<Vbase>V\n%<VLF>pu\n%<angleLF>deg.  SourceProductName=Simscape Electrical
  Mux : Mux  Inputs=10
  Shunt_B106 : powerlib/Elements/Three-Phase Series RLC Load  LConnTagsString=A|B|C  Configuration=Y (grounded)  NominalVoltage=(151009)*1  Vabc=[1e3 1e3 1e3]  Vabcp=[1e3 1e3 1e3]  NominalFrequency=60  UnbalancedPower=off  ActivePower=0  InductivePower=0  CapacitivePower=100e6  Pabc=[10e3 9e3 11e3]  QLabc=[100 90 110]  QCabc=[100 90 110]  Pabcp=[10e3 9e3 11e3]  QLabcp=[100 90 110]  QCabcp=[100 90 110]  Measurements=None  LoadType=constant PQ
      settings: SourceProductName=Simscape Electrical
  W1 : ToWorkspace  VariableName=Q1_3  SampleTime=1/60
  W4 : ToWorkspace  VariableName=P1_3  SampleTime=1/60
  powergui : powerlib/powergui  SimulationMode=Phasor  SampleTime=0  frequency=60  Iterations=50  frequencyindice=60  Pbase=100e6  ErrMax=0.0001  UnitsV=kV  UnitsW=MW  buscounter=0  FunctionMessages=off  echomessages=off  EnableUseOfTLC=off  CurrentSourceSwitches=off  DisableSnubberDevices=off  DisableRonSwitches=off  DisableVfSwitches=off  DisplayEquations=off  AutomaticDiscreteSolvers=off  SolverType=Tustin  Interpol=off  ExternalGateDelay=off  methode=off  Ts=0  x0status=blocks  SPID=off  SwTol=0  HookPort=off  NonlinearTolerance=1e-4  nMaxIteration=100  ContinueOnMaxIteration=off  RestoreLinks=warning  ResistiveCurrentMeasurement=off  Frange=[0:2:500]  Ylog=off  Xlog=on  ShowGrid=off  save=off  variable=ZData  structure=0  ZoomFFT=on  StartTime=0.0  cycles=1  DisplayStyle=1  fundamental=60  FreqAxis=off  MaxFrequency=1000  frequencyindicesteady=1  RmsSteady=1  display=off
      settings: SourceProductName=Simscape Electrical
  pu to Hz : Gain  Gain=60
  w_gen [Hz] : Scope
  123-A : PMIOPort  Side=Right
  123-B : PMIOPort  Port=2  Side=Right
  123-C : PMIOPort  Port=3  Side=Right
  113-A : PMIOPort  Port=4  Side=Right
  113-B : PMIOPort  Port=5  Side=Right
  113-C : PMIOPort  Port=6  Side=Right
  107-A : PMIOPort  Port=7  Side=Right
  107-B : PMIOPort  Port=8  Side=Right
  107-C : PMIOPort  Port=9  Side=Right
  121-A : PMIOPort  Port=10  Side=Left
  121-B : PMIOPort  Port=11  Side=Left
  121-C : PMIOPort  Port=12  Side=Left
  wires:
  [Vabc_B325] -> 3-phase  Instantaneous  Active & Reactive Power/1
  [Iabc_B325] -> 3-phase  Instantaneous  Active & Reactive Power/2
  3-phase  Instantaneous  Active & Reactive Power/1 -> Demux/1
  Demux/1 -> W4/1
  Demux/2 -> W1/1
  [w107] -> Mux/3
  [w118] -> Mux/7
  [w101] -> Mux/1
  [w113] -> Mux/4
  pu to Hz/1 -> w_gen [Hz]/1
  [w116] -> Mux/6
  [w115] -> Mux/5
  [w121] -> Mux/8
  [w122] -> Mux/9
  Mux/1 -> pu to Hz/1
  [w102] -> Mux/2
  [w123] -> Mux/10
  connections:
  A33-2/RConn2 -- A33-1/RConn2 -- 123-B/RConn1 -- B123/RConn2 -- A22/LConn2 -- A21/LConn2
  L105/LConn3 -- B105/RConn3 -- A9/RConn3
  A8/RConn3 -- B104/RConn3 -- L104/LConn3
  A23/LConn1 -- A24/LConn1 -- A28/RConn1 -- A27/RConn1 -- B116/RConn1 -- L116/LConn1
  A23/RConn3 -- A19/LConn3 -- B114/RConn3 -- L114/LConn3
  A25-2/LConn1 -- 121-A/RConn1 -- B121/RConn1 -- A31-1/RConn1 -- A31-2/RConn1 -- A34/RConn1 -- A25-1/LConn1
  A8/RConn1 -- B104/RConn1 -- L104/LConn1
  L107/LConn1 -- B107/RConn1 -- 107-A/RConn1 -- A11/LConn1
  A8/LConn3 -- A12-1/LConn3 -- B109/RConn3 -- L109/LConn3 -- A6/RConn3
  L106/LConn1 -- A10/RConn1 -- Shunt_B106/LConn1 -- B106/RConn1
  A26/LConn2 -- A24/RConn2 -- B115/RConn2 -- L115/LConn2 -- A25-1/RConn2 -- A25-2/RConn2
  B123/RConn1 -- 123-A/RConn1 -- A21/LConn1 -- A33-2/RConn1 -- A33-1/RConn1 -- A22/LConn1
  L120/LConn2 -- A32-2/RConn2 -- A32-3/RConn2 -- B120/RConn2
  L102/LConn3 -- B102/RConn3 -- A1/RConn3 -- A4/RConn3 -- A5/LConn3
  A23/RConn2 -- A19/LConn2 -- B114/RConn2 -- L114/LConn2
  L114/LConn1 -- B114/RConn1 -- A19/LConn1 -- A23/RConn1
  A31-1/RConn2 -- 121-B/RConn1 -- B121/RConn2 -- A25-1/LConn2 -- A25-2/LConn2 -- A34/RConn2 -- A31-2/RConn2
  B116/LConn3 -- 116/RConn3 -- Load Flow Bus7/LConn1
  A5/LConn1 -- A1/RConn1 -- B102/RConn1 -- L102/LConn1 -- A4/RConn1
  B113/RConn1 -- A22/RConn1 -- A20/RConn1 -- A18/RConn1 -- L113/LConn1 -- 113-A/RConn1
  A18/RConn3 -- A22/RConn3 -- A20/RConn3 -- B113/RConn3 -- 113-C/RConn1 -- L113/LConn3
  A32-3/RConn3 -- A32-2/RConn3 -- B120/RConn3 -- L120/LConn3
  A17/LConn1 -- A15/LConn1 -- B112/RConn1
  L118/LConn2 -- A29/LConn2 -- A31-1/LConn2 -- A31-2/LConn2 -- B118/RConn2
  B121/RConn3 -- 121-C/RConn1 -- A34/RConn3 -- A25-2/LConn3 -- A25-1/LConn3 -- A31-1/RConn3 -- A31-2/RConn3
  L102/LConn2 -- B102/RConn2 -- A1/RConn2 -- A4/RConn2 -- A5/LConn2
  A8/LConn1 -- B109/RConn1 -- L109/LConn1 -- A12-1/LConn1 -- A6/RConn1
  A31-2/LConn1 -- A31-1/LConn1 -- A29/LConn1 -- B118/RConn1 -- L118/LConn1
  B110/LConn1 -- A16/RConn1 -- A17/RConn1
  A30/RConn3 -- A27/LConn3 -- B117/RConn3
  A33-2/LConn3 -- A33-1/LConn3 -- B120/LConn3
  L119/LConn3 -- A28/LConn3 -- B119/RConn3
  A13-2/LConn3 -- B110/RConn3 -- L110/LConn3 -- A10/LConn3 -- A9/LConn3
  A19/RConn3 -- A18/LConn3 -- B111/LConn3
  A20/LConn2 -- B112/LConn2 -- A21/RConn2
  A33-1/LConn1 -- B120/LConn1 -- A33-2/LConn1
  A25-2/RConn1 -- A24/RConn1 -- A26/LConn1 -- B115/RConn1 -- L115/LConn1 -- A25-1/RConn1
  A20/LConn3 -- B112/LConn3 -- A21/RConn3
  B121/LConn1 -- 121/RConn1 -- Load Flow Bus1/LConn1
  L103/LConn2 -- B103/RConn2 -- A2/LConn2 -- A6/LConn2
  A23/LConn2 -- A24/LConn2 -- A27/RConn2 -- A28/RConn2 -- B116/RConn2 -- L116/LConn2
  L101/LConn3 -- B101/RConn3 -- A1/LConn3 -- A3/LConn3 -- A2/RConn3
  L105/LConn1 -- B105/RConn1 -- A9/RConn1
  B110/LConn3 -- A16/RConn3 -- A17/RConn3
  L119/LConn2 -- A28/LConn2 -- B119/RConn2
  B122/LConn1 -- 122/RConn1 -- Load Flow Bus10/LConn1
  A34/LConn1 -- A30/LConn1 -- B122/RConn1
  A19/RConn1 -- A18/LConn1 -- B111/LConn1
  A20/LConn1 -- B112/LConn1 -- A21/RConn1
  A19/RConn2 -- A18/LConn2 -- B111/LConn2
  L107/LConn3 -- B107/RConn3 -- 107-C/RConn1 -- A11/LConn3
  A32-2/LConn2 -- B119/LConn2 -- A32-3/LConn2
  A33-1/RConn3 -- 123-C/RConn1 -- B123/RConn3 -- A22/LConn3 -- A21/LConn3 -- A33-2/RConn3
  Load Flow Bus8/LConn1 -- 113/LConn1 -- B113/LConn1
  A32-3/RConn1 -- A32-2/RConn1 -- B120/RConn1 -- L120/LConn1
  B114/LConn1 -- 114/LConn1 -- Load Flow Bus6/LConn1
  A15/RConn2 -- A14/RConn2 -- B109/LConn2
  L101/LConn1 -- A1/LConn1 -- A3/LConn1 -- A2/RConn1 -- B101/RConn1
  A32-3/LConn1 -- B119/LConn1 -- A32-2/LConn1
  L115/LConn3 -- A24/RConn3 -- A26/LConn3 -- A25-1/RConn3 -- A25-2/RConn3 -- B115/RConn3
  A13-2/RConn1 -- A12-1/RConn1 -- B108/RConn1 -- L108/LConn1
  A8/RConn2 -- B104/RConn2 -- L104/LConn2
  A8/LConn2 -- A12-1/LConn2 -- B109/RConn2 -- L109/LConn2 -- A6/RConn2
  A28/RConn3 -- A23/LConn3 -- A24/LConn3 -- L116/LConn3 -- B116/RConn3 -- A27/RConn3
  B119/LConn3 -- A32-2/LConn3 -- A32-3/LConn3
  A34/LConn2 -- A30/LConn2 -- B122/RConn2
  A17/LConn2 -- A15/LConn2 -- B112/RConn2
  B106/RConn2 -- A10/RConn2 -- Shunt_B106/LConn2 -- L106/LConn2
  B101/LConn1 -- 101/LConn1 -- Load Flow Bus2/LConn1
  L101/LConn2 -- A1/LConn2 -- A3/LConn2 -- A2/RConn2 -- B101/RConn2
  B117/RConn2 -- A30/RConn2 -- A27/LConn2
  A6/LConn1 -- B103/RConn1 -- L103/LConn1 -- A2/LConn1
  L110/LConn1 -- A10/LConn1 -- A9/LConn1 -- A13-2/LConn1 -- B110/RConn1
  L113/LConn2 -- A22/RConn2 -- A20/RConn2 -- A18/RConn2 -- B113/RConn2 -- 113-B/RConn1
  B117/RConn1 -- A30/RConn1 -- A27/LConn1
  L118/LConn3 -- A29/LConn3 -- A31-1/LConn3 -- A31-2/LConn3 -- B118/RConn3
  A15/RConn3 -- A14/RConn3 -- B109/LConn3
  A34/LConn3 -- A30/LConn3 -- B122/RConn3
  B118/LConn1 -- 118/RConn1 -- Load Flow Bus/LConn1
  B115/LConn3 -- 115/RConn3 -- Load Flow Bus5/LConn1
  B111/RConn3 -- A16/LConn3 -- A14/LConn3
  B111/RConn2 -- A16/LConn2 -- A14/LConn2
  B102/LConn1 -- 102/LConn1 -- Load Flow Bus3/LConn1
  L108/LConn3 -- A12-1/RConn3 -- A13-2/RConn3 -- B108/RConn3
  L105/LConn2 -- B105/RConn2 -- A9/RConn2
  A33-1/LConn2 -- B120/LConn2 -- A33-2/LConn2
  L103/LConn3 -- B103/RConn3 -- A2/LConn3 -- A6/LConn3
  B107/LConn1 -- 107/LConn1 -- Load Flow Bus4/LConn1
  L119/LConn1 -- A28/LConn1 -- B119/RConn1
  B110/LConn2 -- A16/RConn2 -- A17/RConn2
  A15/RConn1 -- A14/RConn1 -- B109/LConn1
  Shunt_B106/LConn3 -- A10/RConn3 -- L106/LConn3 -- B106/RConn3
  B111/RConn1 -- A16/LConn1 -- A14/LConn1
  A13-2/LConn2 -- A10/LConn2 -- A9/LConn2 -- B110/RConn2 -- L110/LConn2
  L107/LConn2 -- B107/RConn2 -- 107-B/RConn1 -- A11/LConn2
  A17/LConn3 -- A15/LConn3 -- B112/RConn3
  L108/LConn2 -- A12-1/RConn2 -- A13-2/RConn2 -- B108/RConn2
  Load Flow Bus9/LConn1 -- 123/LConn1 -- B123/LConn1
  122/RConn3 -- B122/LConn3
  A29/RConn1 -- B117/LConn1
  B108/LConn3 -- A11/RConn3
  A4/LConn3 -- B104/LConn3
  B108/LConn2 -- A11/RConn2
  A5/RConn3 -- B106/LConn3
  A5/RConn1 -- B106/LConn1
  114/LConn3 -- B114/LConn3
  A3/RConn1 -- B105/LConn1
  123/LConn3 -- B123/LConn3
  115/RConn1 -- B115/LConn1
  113/LConn2 -- B113/LConn2
  B124/LConn3 -- A26/RConn3
  B124/LConn1 -- A26/RConn1
  A29/RConn3 -- B117/LConn3
  A29/RConn2 -- B117/LConn2
  B124/LConn2 -- A26/RConn2
  A7/LConn1 -- B124/RConn1
  B103/LConn3 -- A7/RConn3
  A3/RConn2 -- B105/LConn2
  B103/LConn2 -- A7/RConn2
  B103/LConn1 -- A7/RConn1
  A7/LConn2 -- B124/RConn2
  A5/RConn2 -- B106/LConn2
  A4/LConn1 -- B104/LConn1
  B104/LConn2 -- A4/LConn2
  121/RConn2 -- B121/LConn2
  116/RConn1 -- B116/LConn1
  118/RConn2 -- B118/LConn2
  121/RConn3 -- B121/LConn3
  115/RConn2 -- B115/LConn2
  113/LConn3 -- B113/LConn3
  116/RConn2 -- B116/LConn2
  B108/LConn1 -- A11/RConn1
  107/LConn3 -- B107/LConn3
  102/LConn2 -- B102/LConn2
  102/LConn3 -- B102/LConn3
  A7/LConn3 -- B124/RConn3
  122/RConn2 -- B122/LConn2
  101/LConn3 -- B101/LConn3
  101/LConn2 -- B101/LConn2
  107/LConn2 -- B107/LConn2
  118/RConn3 -- B118/LConn3
  123/LConn2 -- B123/LConn2
  114/LConn2 -- B114/LConn2
  A3/RConn3 -- B105/LConn3
